simulink model "pidLoopTestDUT"  (R2017a)
settings: Solver=VariableStepAuto  StartTime=0.0  StopTime=inf  RelTol=1e-3
libraries: simulink x1
settings Model: Creator=Nicoe Welch  LastModifiedBy=Nicoe Welch

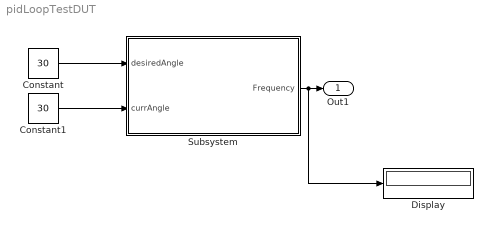
== system pidLoopTestDUT ==
  Constant : Constant  Value=30
  Constant1 : Constant  Value=30
  Display : Display
  Subsystem : Subsystem
  Out1 : Outport
  wires:
  Constant/1 -> Subsystem/1(desiredAngle)
  Constant1/1 -> Subsystem/2(currAngle)
  Subsystem/1(Frequency) -> Display/1, Out1/1

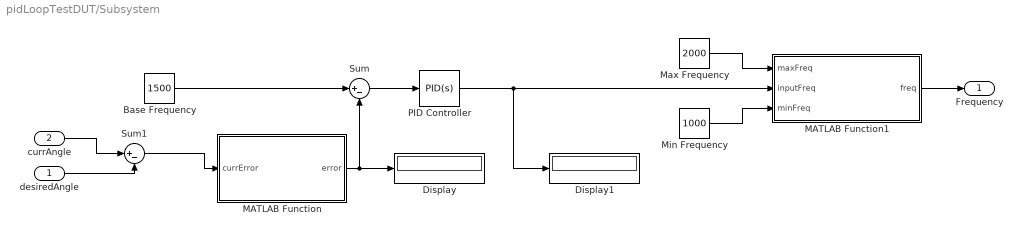
== system pidLoopTestDUT/Subsystem ==
  desiredAngle : Inport
  currAngle : Inport  Port=2
  Base Frequency : Constant  Value=1500
  Display : Display
  Display1 : Display
  MATLAB Function : MATLAB Function  TreatAsAtomicUnit=on
  MATLAB Function1 : MATLAB Function  TreatAsAtomicUnit=on
  Max Frequency : Constant  Value=2000
  Min Frequency : Constant  Value=1000
  PID Controller : simulink/Continuous/PID Controller  Controller=PID  TimeDomain=Continuous-time  SampleTime=-1  IntegratorMethod=Forward Euler  FilterMethod=Forward Euler  Form=Parallel  UseFilter=on  ControllerParametersSource=internal  P=1  I=0  D=0  N=100  InitialConditionSource=internal  InitialConditionForIntegrator=0  InitialConditionForFilter=0  ExternalReset=none  LimitOutput=off  UpperSaturationLimit=inf  LowerSaturationLimit=-inf  LinearizeAsGain=on  AntiWindupMode=none  Kb=1  TrackingMode=off  Kt=1  PParamMin=[]  PParamMax=[]  IParamMin=[]  IParamMax=[]  DParamMin=[]  DParamMax=[]  NParamMin=[]  NParamMax=[]  KbParamMin=[]  KbParamMax=[]  KtParamMin=[]  KtParamMax=[]  POutMin=[]  POutMax=[]  IOutMin=[]  IOutMax=[]  DOutMin=[]  DOutMax=[]  NOutMin=[]  NOutMax=[]  KbOutMin=[]  KbOutMax=[]  KtOutMin=[]  KtOutMax=[]  IntegratorOutMin=[]  IntegratorOutMax=[]  FilterOutMin=[]  FilterOutMax=[]  SumOutMin=[]  SumOutMax=[]  SumI1OutMin=[]  SumI1OutMax=[]  SumI2OutMin=[]  SumI2OutMax=[]  SumI3OutMin=[]  SumI3OutMax=[]  SumDOutMin=[]  SumDOutMax=[]  SaturationOutMin=[]  SaturationOutMax=[]  IntegratorContinuousStateAttributes=''  IntegratorStateMustResolveToSignalObject=off  IntegratorRTWStateStorageClass=Auto  FilterContinuousStateAttributes=''  FilterStateMustResolveToSignalObject=off  FilterRTWStateStorageClass=Auto  DifferentiatorICPrevScaledInput=0  DifferentiatorOutMin=[]  DifferentiatorOutMax=[]  InitialConditionSetting=State (most efficient)
  Sum : Sum  Inputs=|+-
  Sum1 : Sum  Inputs=|+-
  Frequency : Outport
  wires:
  Sum/1 -> PID Controller/1
  Base Frequency/1 -> Sum/1
  MATLAB Function1/1(freq) -> Frequency/1
  Min Frequency/1 -> MATLAB Function1/3(minFreq)
  Max Frequency/1 -> MATLAB Function1/1(maxFreq)
  PID Controller/1 -> Display1/1, MATLAB Function1/2(inputFreq)
  desiredAngle/1 -> Sum1/2
  currAngle/1 -> Sum1/1
  MATLAB Function/1(error) -> Display/1, Sum/2
  Sum1/1 -> MATLAB Function/1(currError)

== matlab function pidLoopTestDUT/Subsystem/MATLAB Function ==
  data: error output; currError input
function error = fcn(currError)
transError = -.01080*(currError)^3 + .678*(currError)^2 + 2.124*(currError) + 22.653;
if currError < 0
    error = transError * -1;
else
    error = transError;
end

== matlab function pidLoopTestDUT/Subsystem/MATLAB Function1 ==
  data: maxFreq input; inputFreq input; freq output; minFreq input
function freq = fcn(maxFreq,inputFreq, minFreq)
    if( inputFreq > maxFreq ) 
        freq = maxFreq
    elseif ( inputFreq < minFreq ) 
        freq = minFreq
    else 
        freq = inputFreq
    end
